simulink model "xdot_obac"  (Simulink 7.2)
settings: Solver=FixedStepDiscrete  StartTime=0.0  StopTime=0  FixedStep=MACH.dt  RelTol=1e-3
undefined symbols (not defined in the file or in its folder): MACH, MACH_mass_IC, obac_params
libraries: model_lib x3, models x1
settings Model: Creator=E183308  LastModifiedBy=E183308  BufferReuse=off
settings DataIOCC: ExternalInput=[0 xu]  InitialState=[]  LoadExternalInput=on  LoadInitialState=on  SaveOutput=off  SaveTime=off  SignalLoggingName=sigsOut
settings OptimizationCC: InlineParams=on  BufferReuse=off  InitFltsAndDblsToZero=on
settings DebuggingCC: SaveWithParameterizedLinksMsg=none  SignalResolutionControl=TryResolveAllWithWarning  SolverPrmCheckMsg=none  InheritedTsInSrcMsg=none  MultiTaskDSMMsg=warning  MultiTaskCondExecSysMsg=none  StrictBusMsg=None
settings HardwareCC: TargetUnknown=on
settings RTWCC: IncludeERTFirstTime=on
settings GRTTargetCC: TargetFcnLib=ansi_tfl_tmw.mat

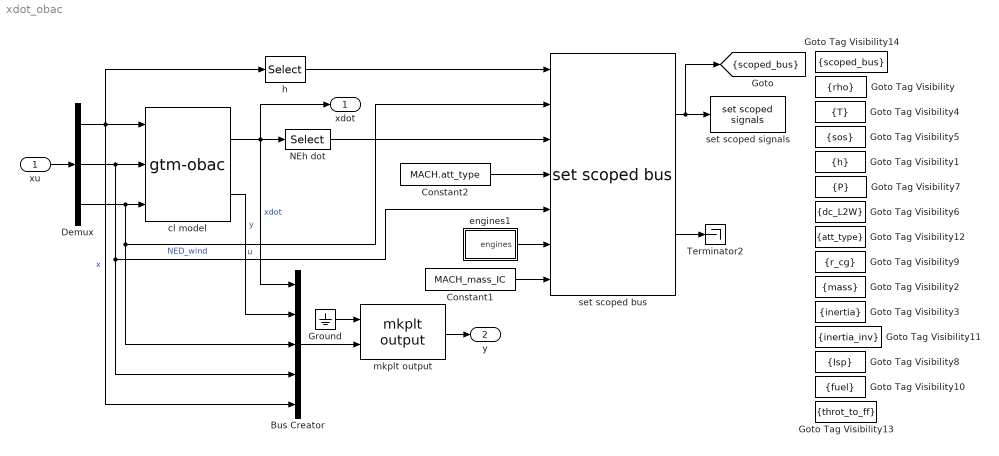
== system xdot_obac ==
  xu : Inport  OutDataType=sfix(16)  OutScaling=2^0
  Bus Creator : BusCreator  Inputs=5
  Constant1 : Constant  Value=MACH_mass_IC  OutDataType=sfix(16)  OutScaling=2^0
  Constant2 : Constant  Value=MACH.att_type  OutDataType=sfix(16)  OutScaling=2^0
  Demux : Demux  Outputs=[MACH.num_x MACH.num_u 3]
  Goto Tag Visibility : GotoTagVisibility  GotoTag=rho
  Goto Tag Visibility1 : GotoTagVisibility  GotoTag=h
  Goto Tag Visibility10 : GotoTagVisibility  GotoTag=fuel
  Goto Tag Visibility11 : GotoTagVisibility  GotoTag=inertia_inv
  Goto Tag Visibility12 : GotoTagVisibility  GotoTag=att_type
  Goto Tag Visibility13 : GotoTagVisibility  GotoTag=throt_to_ff
  Goto Tag Visibility14 : GotoTagVisibility  GotoTag=scoped_bus
  Goto Tag Visibility2 : GotoTagVisibility  GotoTag=mass
  Goto Tag Visibility3 : GotoTagVisibility  GotoTag=inertia
  Goto Tag Visibility4 : GotoTagVisibility  GotoTag=T
  Goto Tag Visibility5 : GotoTagVisibility  GotoTag=sos
  Goto Tag Visibility6 : GotoTagVisibility  GotoTag=dc_L2W
  Goto Tag Visibility7 : GotoTagVisibility  GotoTag=P
  Goto Tag Visibility8 : GotoTagVisibility  GotoTag=Isp
  Goto Tag Visibility9 : GotoTagVisibility  GotoTag=r_cg
  Ground : Ground
  NEh dot : Selector  InputPortWidth=obac_params.num_x  IndexOptions=Index vector (dialog)  Indices=MACH.NEh_idx  OutputSizes=1
  Terminator2 : Terminator
  cl model : models/gtm-obac  SystemSampleTime=-1
  engines1 : Subsystem
  h : Selector  InputPortWidth=obac_params.num_x  IndexOptions=Index vector (dialog)  Indices=MACH.NEh_idx(3)  OutputSizes=1
  mkplt output : model_lib/mkplt output  SystemSampleTime=-1
  set scoped bus : model_lib/set scoped bus  SystemSampleTime=-1  vehicle_params=obac_params
  set scoped signals : model_lib/set scoped signals  SystemSampleTime=-1
  xdot : Outport  OutDataType=sfix(16)  OutScaling=2^0
  y : Outport  Port=2  OutDataType=sfix(16)  OutScaling=2^0
  tag scope: scoped_bus=scoped
  wires:
  Demux/1 -> cl model/1, h/1, Bus Creator/5  "x"
  Demux/2 -> cl model/2, set scoped bus/5, Bus Creator/4  "u"
  Demux/3 -> cl model/3, set scoped bus/2, Bus Creator/3  "NED_wind"
  xu/1 -> Demux/1
  cl model/1 -> xdot/1, NEh dot/1, Bus Creator/1  "xdot"
  h/1 -> set scoped bus/1
  NEh dot/1 -> set scoped bus/3
  Constant2/1 -> set scoped bus/4
  set scoped bus/1 -> set scoped signals/1, [scoped_bus]
  set scoped bus/2 -> Terminator2/1
  mkplt output/1 -> y/1
  Ground/1 -> mkplt output/1
  Bus Creator/1 -> mkplt output/2
  cl model/2 -> Bus Creator/2  "y"
  Constant1/1 -> set scoped bus/7
  engines1/1(engines) -> set scoped bus/6

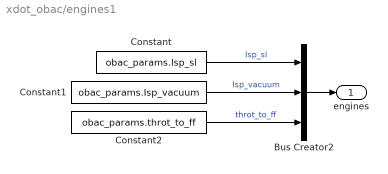
== system xdot_obac/engines1 ==
  Bus Creator2 : BusCreator  Inputs=3
  Constant : Constant  Value=obac_params.Isp_sl  OutDataType=sfix(16)  OutScaling=2^0
  Constant1 : Constant  Value=obac_params.Isp_vacuum  OutDataType=sfix(16)  OutScaling=2^0
  Constant2 : Constant  Value=obac_params.throt_to_ff  OutDataType=sfix(16)  OutScaling=2^0
  engines : Outport  OutDataType=sfix(16)  OutScaling=2^0
  wires:
  Constant1/1 -> Bus Creator2/2  "Isp_vacuum"
  Constant/1 -> Bus Creator2/1  "Isp_sl"
  Bus Creator2/1 -> engines/1
  Constant2/1 -> Bus Creator2/3  "throt_to_ff"
